simulink model "motor_idle"  (R2025b)
settings: Solver=ode45  StartTime=0.0  StopTime=10  MaxStep=0.02  RelTol=1e-3  AbsTol=1e-3
values from neighbouring files (symbols this model uses):
  B = 0.072    [parametros.m]
  Cd = 0.7    [parametros.m]
  emax = 1.8    [parametros.m]
  Hl = 44e6    (= 44000000)    [parametros.m]
  J = 0.25    [parametros.m]
  k1 = 1.44e5    (= 144000)    [parametros.m]
  k2 = 0.46    [parametros.m]
  k3 = 9.1e-4    (= 0.00091)    [parametros.m]
  k4 = 0.075    [parametros.m]
  kappa = 1.4    [parametros.m]
  kqueda = 0.001    [parametros.m]
  N0 = 800    [parametros.m]
  N_ciclo = 2    [parametros.m]
  nVol = 0.85    [parametros.m]
  omega0 = N0 * 2*pi/60    (= 83.7758040957)    [parametros.m]
  P_atm = 101325    [parametros.m]
  Pim0 = 40000    [parametros.m]
  R = 287    [parametros.m]
  S = 0.0814    [parametros.m]
  SA = 20    [parametros.m]
  SA_MBT = 25    [parametros.m]
  sigma0 = 14.7    [parametros.m]
  T_im = 300    [parametros.m]
  V = 0.0015    [parametros.m]
  V_d = 0.0013    [parametros.m]
settings Model: Creator=thiag  LastModifiedBy=thiag

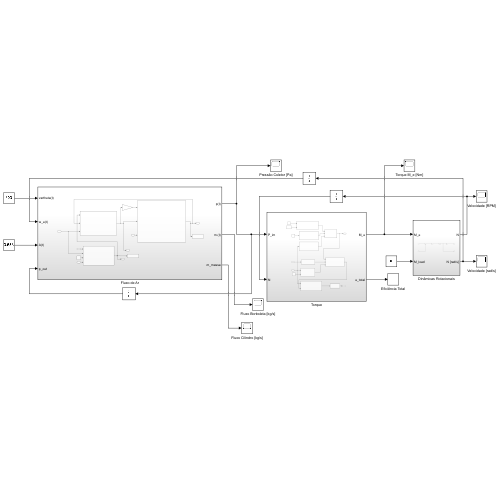
[thumbnail: Simulink's stored preview of the top-level diagram]
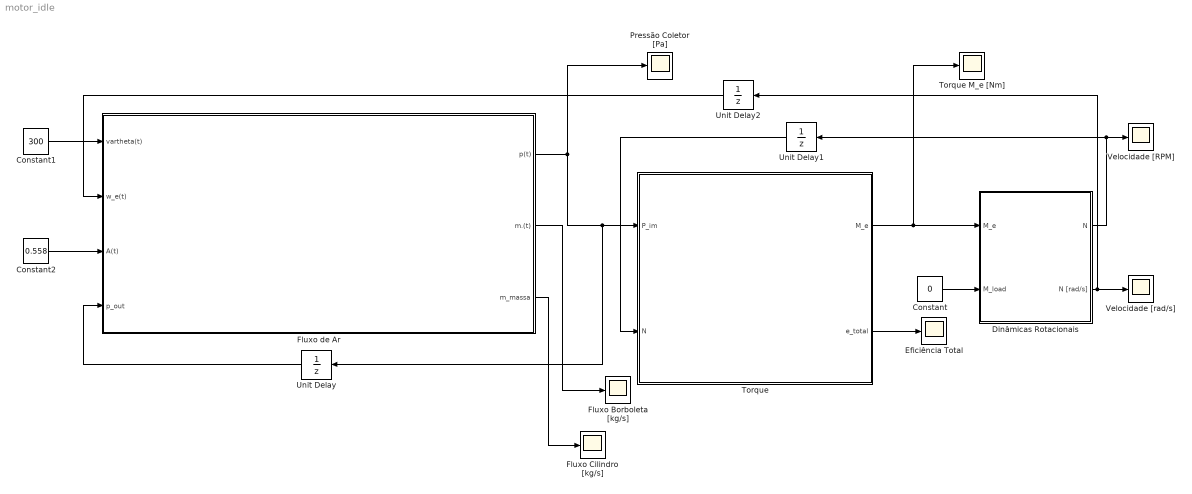
== system motor_idle ==
  Constant : Constant  Value=0
  Constant1 : Constant  Value=300
  Constant2 : Constant  Value=0.558
  Dinâmicas Rotacionais : Subsystem
  Eficiência Total : Scope
      settings: ActiveDisplayYMinimum=0.27237825090968576  ActiveDisplayYMaximum=0.32200698501713004  DataLoggingVariableName=ScopeData2
  Fluxo Borboleta [kg/s] : Scope
      settings: ActiveDisplayYMinimum=0.00082356518942528151  ActiveDisplayYMaximum=0.0010235651894252816  DataLoggingVariableName=ScopeData5
  Fluxo Cilindro [kg/s] : Scope
      settings: ActiveDisplayYMinimum=0.00036149983076327858  ActiveDisplayYMaximum=0.0037240393540282214  DataLoggingVariableName=ScopeData6
  Fluxo de Ar : Subsystem
  Pressão Coletor [Pa] : Scope
      settings: ActiveDisplayYMinimum=7090.5549569777586  ActiveDisplayYMaximum=43656.605004780249  DataLoggingVariableName=ScopeData3
  Torque : Subsystem
  Torque M_e [Nm] : Scope
      settings: ActiveDisplayYMinimum=-87.316847243549518  ActiveDisplayYMaximum=243.76291501335962  DataLoggingVariableName=ScopeData4
  Unit Delay : UnitDelay  InitialCondition=Pim0  SampleTime=0.02  HasFrameUpgradeWarning=on
  Unit Delay1 : UnitDelay  InitialCondition=N0  SampleTime=0.02  HasFrameUpgradeWarning=on
  Unit Delay2 : UnitDelay  InitialCondition=omega0  SampleTime=0.02  HasFrameUpgradeWarning=on
  Velocidade [RPM] : Scope
      settings: ActiveDisplayYMinimum=398.86041068334004  ActiveDisplayYMaximum=1697.6811601075797
  Velocidade [rad/s] : Scope
      settings: ActiveDisplayYMinimum=55.585400826373068  ActiveDisplayYMaximum=178.72399012064108
  wires:
  Dinâmicas Rotacionais/2(N [rad/s]) -> Velocidade [rad/s]/1, Unit Delay2/1
  Dinâmicas Rotacionais/1(N) -> Unit Delay1/1, Velocidade [RPM]/1
  Torque/2(e_total) -> Eficiência Total/1
  Torque/1(M_e) -> Torque M_e [Nm]/1, Dinâmicas Rotacionais/1(M_e)
  Fluxo de Ar/1(p(t)) -> Unit Delay/1, Torque/1(P_im), Pressão Coletor [Pa]/1
  Constant/1 -> Dinâmicas Rotacionais/2(M_load)
  Constant1/1 -> Fluxo de Ar/1(vartheta(t))
  Constant2/1 -> Fluxo de Ar/3(A(t))
  Fluxo de Ar/2(m.(t)) -> Fluxo Borboleta [kg/s]/1
  Fluxo de Ar/3(m_massa) -> Fluxo Cilindro [kg/s]/1
  Unit Delay/1 -> Fluxo de Ar/4(p_out)
  Unit Delay2/1 -> Fluxo de Ar/2(w_e(t))
  Unit Delay1/1 -> Torque/2(N)

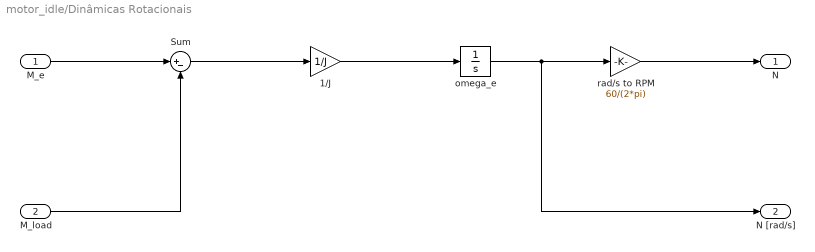
== system motor_idle/Dinâmicas Rotacionais ==
  M_e : Inport
  M_load : Inport  Port=2
  1/J : Gain  Gain=1/J
  Sum : Sum  Inputs=|+-
  omega_e : Integrator  InitialCondition=(N0*2*pi)/60
  rad/s to RPM : Gain  Gain=60/(2*pi)
  N : Outport
  N [rad/s] : Outport  Port=2
  wires:
  M_e/1 -> Sum/1
  M_load/1 -> Sum/2
  Sum/1 -> 1/J/1
  1/J/1 -> omega_e/1
  omega_e/1 -> N [rad/s]/1, rad/s to RPM/1
  rad/s to RPM/1 -> N/1

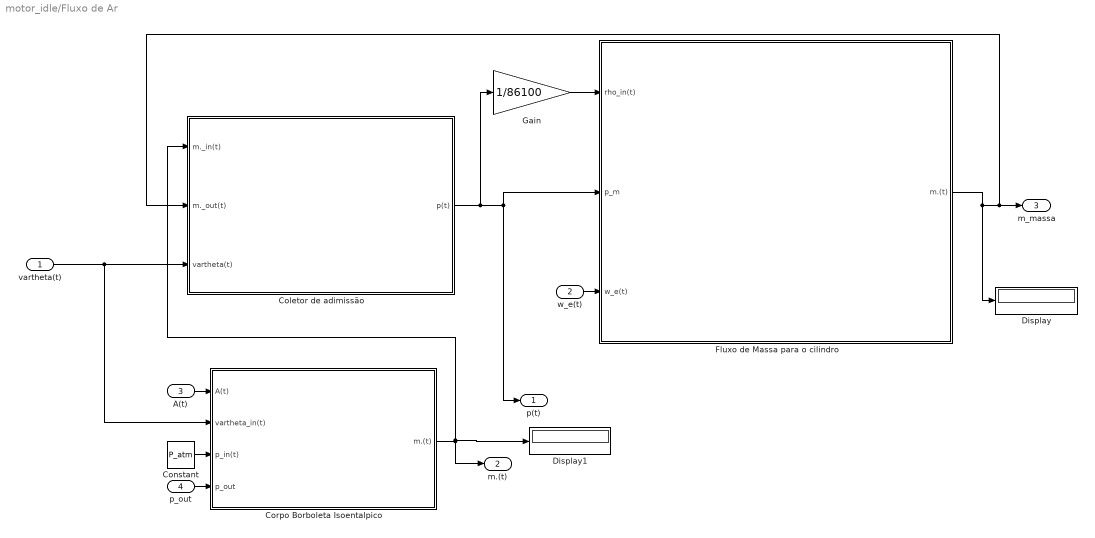
== system motor_idle/Fluxo de Ar ==
  vartheta(t) : Inport
  w_e(t) : Inport  Port=2
  A(t) : Inport  Port=3
  p_out : Inport  Port=4
  Coletor de adimissão : Subsystem
  Constant : Constant  Value=P_atm
  Corpo Borboleta Isoentalpico : Subsystem
  Display : Display
  Display1 : Display
  Fluxo de Massa para o cilindro : Subsystem
  Gain : Gain  Gain=1/86100
  p(t) : Outport
  m.(t) : Outport  Port=2
  m_massa : Outport  Port=3
  wires:
  Coletor de adimissão/1(p(t)) -> p(t)/1, Fluxo de Massa para o cilindro/2(p_m), Gain/1
  Constant/1 -> Corpo Borboleta Isoentalpico/3(p_in(t))
  Corpo Borboleta Isoentalpico/1(m.(t)) -> m.(t)/1, Display1/1, Coletor de adimissão/1(m._in(t))
  p_out/1 -> Corpo Borboleta Isoentalpico/4(p_out)
  w_e(t)/1 -> Fluxo de Massa para o cilindro/3(w_e(t))
  Fluxo de Massa para o cilindro/1(m.(t)) -> Display/1, m_massa/1, Coletor de adimissão/2(m._out(t))
  A(t)/1 -> Corpo Borboleta Isoentalpico/1(A(t))
  vartheta(t)/1 -> Corpo Borboleta Isoentalpico/2(vartheta_in(t)), Coletor de adimissão/3(vartheta(t))
  Gain/1 -> Fluxo de Massa para o cilindro/1(rho_in(t))

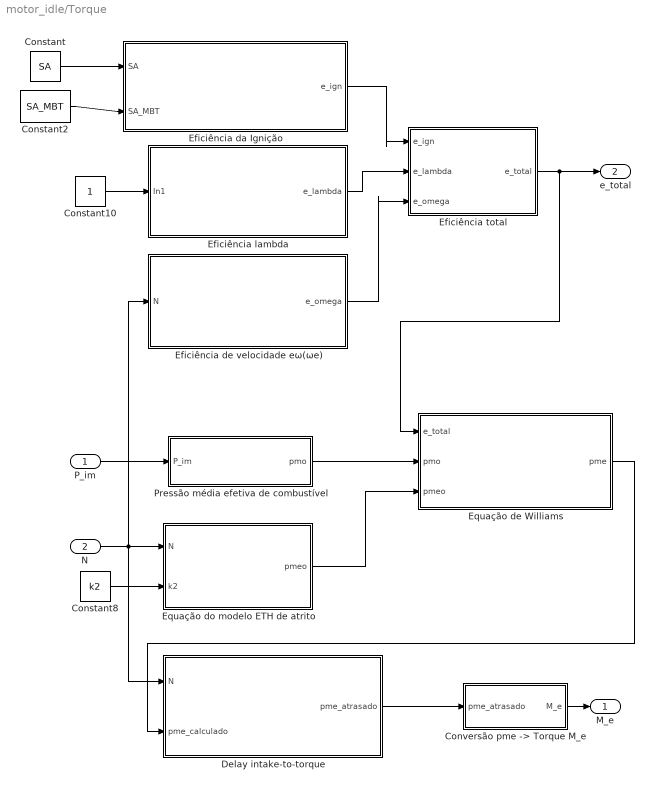
== system motor_idle/Torque ==
  P_im : Inport
  N : Inport  Port=2
  Constant : Constant  Value=SA
  Constant10 : Constant
  Constant2 : Constant  Value=SA_MBT
  Constant8 : Constant  Value=k2
  "Conversão pme -> Torque M_e" : Subsystem
  Delay intake-to-torque : Subsystem
  Eficiência da Ignição : Subsystem
  Eficiência de velocidade eω(ωe) : Subsystem
  Eficiência lambda : Subsystem
  Eficiência total : Subsystem
  Equação de Williams : Subsystem
  Equação do modelo ETH de atrito : Subsystem
  Pressão média efetiva de combustível : Subsystem
  M_e : Outport
  e_total : Outport  Port=2
  wires:
  N/1 -> Delay intake-to-torque/1(N), Eficiência de velocidade eω(ωe)/1(N), Equação do modelo ETH de atrito/1(N)
  Eficiência de velocidade eω(ωe)/1(e_omega) -> Eficiência total/3(e_omega)
  Constant/1 -> Eficiência da Ignição/1(SA)
  Equação do modelo ETH de atrito/1(pmeo) -> Equação de Williams/3(pmeo)
  Constant2/1 -> Eficiência da Ignição/2(SA_MBT)
  P_im/1 -> Pressão média efetiva de combustível/1(P_im)
  Equação de Williams/1(pme) -> Delay intake-to-torque/2(pme_calculado)
  Eficiência lambda/1(e_lambda) -> Eficiência total/2(e_lambda)
  Pressão média efetiva de combustível/1(pmo) -> Equação de Williams/2(pmo)
  Constant8/1 -> Equação do modelo ETH de atrito/2(k2)
  Constant10/1 -> Eficiência lambda/1(In1)
  Delay intake-to-torque/1(pme_atrasado) -> "Conversão pme -> Torque M_e"/1(pme_atrasado)
  Eficiência da Ignição/1(e_ign) -> Eficiência total/1(e_ign)
  Eficiência total/1(e_total) -> e_total/1, Equação de Williams/1(e_total)
  "Conversão pme -> Torque M_e"/1(M_e) -> M_e/1

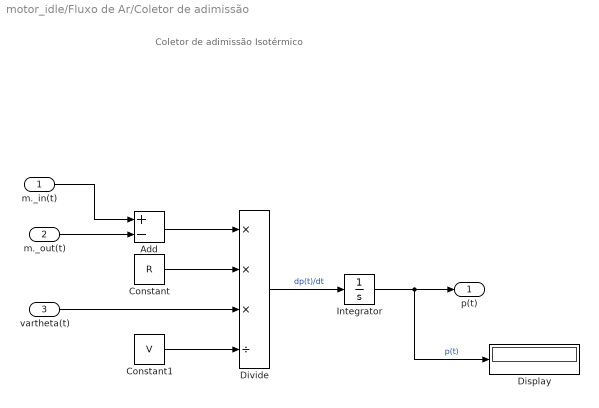
== system motor_idle/Fluxo de Ar/Coletor de adimissão ==
  note: Coletor de adimissão Isotérmico
  m._in(t) : Inport
  m._out(t) : Inport  Port=2
  vartheta(t) : Inport  Port=3
  Add : Sum  Inputs=+-
  Constant : Constant  Value=R
  Constant1 : Constant  Value=V
  Display : Display
  Divide : Product  Inputs=***/
  Integrator : Integrator  InitialCondition=Pim0
  p(t) : Outport
  wires:
  Add/1 -> Divide/1
  Constant/1 -> Divide/2
  m._in(t)/1 -> Add/1
  Divide/1 -> Integrator/1  "dp(t)/dt"
  Constant1/1 -> Divide/4
  m._out(t)/1 -> Add/2
  Integrator/1 -> Display/1, p(t)/1  "p(t)"
  vartheta(t)/1 -> Divide/3

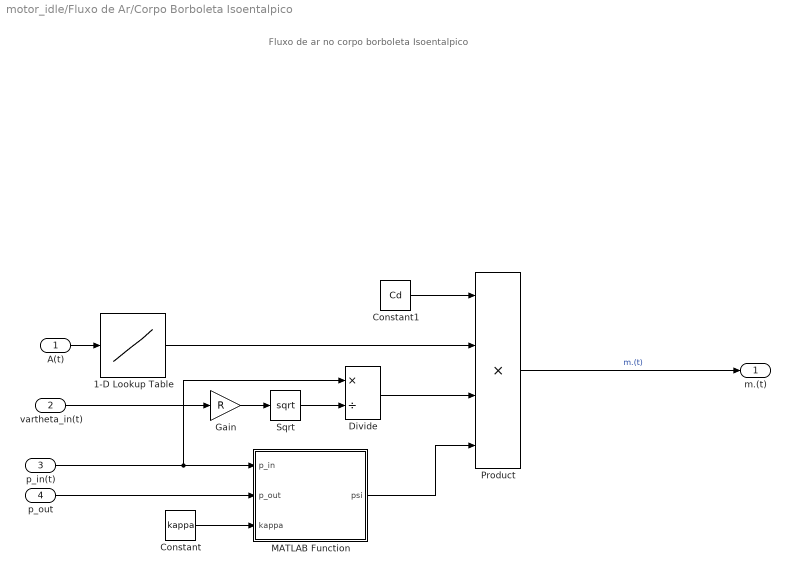
== system motor_idle/Fluxo de Ar/Corpo Borboleta Isoentalpico ==
  note: Fluxo de ar no corpo borboleta Isoentalpico
  A(t) : Inport
  vartheta_in(t) : Inport  Port=2
  p_in(t) : Inport  Port=3
  p_out : Inport  Port=4
  1-D Lookup Table : Lookup_n-D  NumberOfTableDimensions=1  BreakpointsForDimension1=[0, 5, 10, 20, 45, 90]  Table=[0, 5e-5, 1e-4, 2e-4, 3.5e-4, 5e-4]  InternalRulePriority=Speed  RndMeth=Simplest
  Constant : Constant  Value=kappa
  Constant1 : Constant  Value=Cd
  Divide : Product  Inputs=*/
  Gain : Gain  Gain=R
  MATLAB Function : MATLAB Function  TreatAsAtomicUnit=on
  Product : Product  Inputs=4
  Sqrt : Sqrt
  m.(t) : Outport
  wires:
  Constant/1 -> MATLAB Function/3(kappa)
  MATLAB Function/1(psi) -> Product/4
  p_in(t)/1 -> Divide/1, MATLAB Function/1(p_in)
  Sqrt/1 -> Divide/2
  Gain/1 -> Sqrt/1
  Divide/1 -> Product/3
  Constant1/1 -> Product/1
  Product/1 -> m.(t)/1  "m.(t)"
  vartheta_in(t)/1 -> Gain/1
  p_out/1 -> MATLAB Function/2(p_out)
  1-D Lookup Table/1 -> Product/2
  A(t)/1 -> 1-D Lookup Table/1

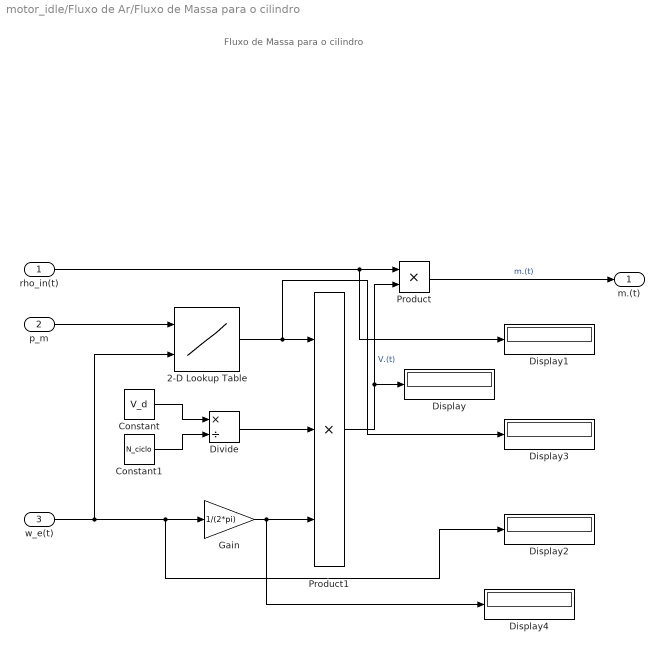
== system motor_idle/Fluxo de Ar/Fluxo de Massa para o cilindro ==
  note: Fluxo de Massa para o cilindro
  rho_in(t) : Inport
  p_m : Inport  Port=2
  w_e(t) : Inport  Port=3
  2-D Lookup Table : Lookup_n-D  BreakpointsForDimension1=[20000, 40000, 60000, 80000, 101325]  BreakpointsForDimension2=[52, 83, 105, 157, 209]  Table=[0.60 0.62 0.63 0.65 0.66; 0.75 0.78 0.80 0.82 0.83; 0.82 0.84 0.85 0.86 0.87; 0.85 0.86 0.87 0.88 0.89; 0.87 0.88 0.89 0.90 0.91]  InternalRulePriority=Speed  RndMeth=Simplest
      settings: InputPortMap=u0,u1
  Constant : Constant  Value=V_d
  Constant1 : Constant  Value=N_ciclo
  Display{,1..4} (5 alike) : Display
  Divide : Product  Inputs=*/
  Gain : Gain  Gain=1/(2*pi)
  Product : Product
  Product1 : Product  Inputs=3
  m.(t) : Outport
  wires:
  rho_in(t)/1 -> Display1/1, Product/1
  Product1/1 -> Display/1, Product/2  "V.(t)"
  p_m/1 -> 2-D Lookup Table/1
  Constant1/1 -> Divide/2
  Constant/1 -> Divide/1
  Gain/1 -> Display4/1, Product1/3
  Divide/1 -> Product1/2
  2-D Lookup Table/1 -> Display3/1, Product1/1
  Product/1 -> m.(t)/1  "m.(t)"
  w_e(t)/1 -> 2-D Lookup Table/2, Display2/1, Gain/1

== system motor_idle/Torque/Conversão pme -> Torque M_e ==
  pme_atrasado : Inport
  Gain7 : Gain  Gain=V_d/4*pi
  M_e : Outport
  wires:
  Gain7/1 -> M_e/1
  pme_atrasado/1 -> Gain7/1

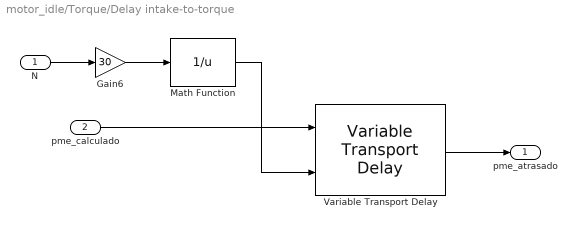
== system motor_idle/Torque/Delay intake-to-torque ==
  N : Inport
  pme_calculado : Inport  Port=2
  Gain6 : Gain  Gain=30
  Math Function : Math  Operator=reciprocal
  Variable Transport Delay : VariableTransportDelay  VariableDelayType=Variable transport delay  MaximumDelay=0.1  MaximumPoints=8192
  pme_atrasado : Outport
  wires:
  pme_calculado/1 -> Variable Transport Delay/1
  N/1 -> Gain6/1
  Gain6/1 -> Math Function/1
  Math Function/1 -> Variable Transport Delay/2
  Variable Transport Delay/1 -> pme_atrasado/1

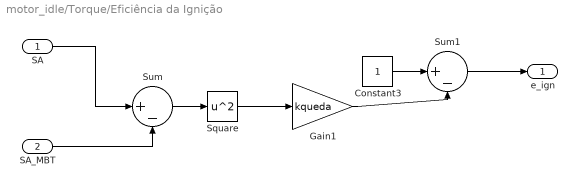
== system motor_idle/Torque/Eficiência da Ignição ==
  SA : Inport
  SA_MBT : Inport  Port=2
  Constant3 : Constant
  Gain1 : Gain  Gain=kqueda
  Square : Math  Operator=square
  Sum : Sum  Inputs=|+-
  Sum1 : Sum  Inputs=|+-
  e_ign : Outport
  wires:
  Gain1/1 -> Sum1/2
  Sum1/1 -> e_ign/1
  Constant3/1 -> Sum1/1
  SA/1 -> Sum/1
  SA_MBT/1 -> Sum/2
  Square/1 -> Gain1/1
  Sum/1 -> Square/1

== system motor_idle/Torque/Eficiência de velocidade eω(ωe) ==
  N : Inport
  1-D Lookup Table1 : Lookup_n-D  NumberOfTableDimensions=1  BreakpointsForDimension1="[52,  83,  105, 157, 209, 262, 314, 419, 524, 628]"  Table=[0.28, 0.30, 0.31, 0.33, 0.34, 0.35, 0.35, 0.34, 0.32, 0.29]  InternalRulePriority=Speed  RndMeth=Simplest
  Gain2 : Gain  Gain=(2*pi)/60
  e_omega : Outport
  wires:
  N/1 -> Gain2/1
  1-D Lookup Table1/1 -> e_omega/1
  Gain2/1 -> 1-D Lookup Table1/1

== system motor_idle/Torque/Eficiência lambda ==
  In1 : Inport
  1-D Lookup Table : Lookup_n-D  NumberOfTableDimensions=1  BreakpointsForDimension1=[0.70, 0.80, 0.90, 0.95, 1.00, 1.03, 1.10, 1.30]  Table=[0.59, 0.72, 0.86, 0.93, 0.98, 1.00, 1.00, 1.00]  InternalRulePriority=Speed  RndMeth=Simplest
  e_lambda : Outport
  wires:
  In1/1 -> 1-D Lookup Table/1
  1-D Lookup Table/1 -> e_lambda/1

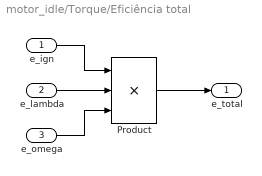
== system motor_idle/Torque/Eficiência total ==
  e_ign : Inport
  e_lambda : Inport  Port=2
  e_omega : Inport  Port=3
  Product : Product  Inputs=3
  e_total : Outport
  wires:
  Product/1 -> e_total/1
  e_omega/1 -> Product/3
  e_lambda/1 -> Product/2
  e_ign/1 -> Product/1

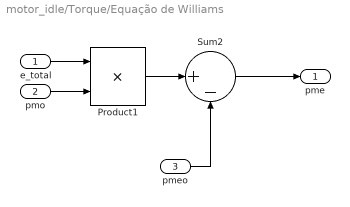
== system motor_idle/Torque/Equação de Williams ==
  e_total : Inport
  pmo : Inport  Port=2
  pmeo : Inport  Port=3
  Product1 : Product
  Sum2 : Sum  Inputs=|+-
  pme : Outport
  wires:
  Product1/1 -> Sum2/1
  Sum2/1 -> pme/1
  pmeo/1 -> Sum2/2
  e_total/1 -> Product1/1
  pmo/1 -> Product1/2

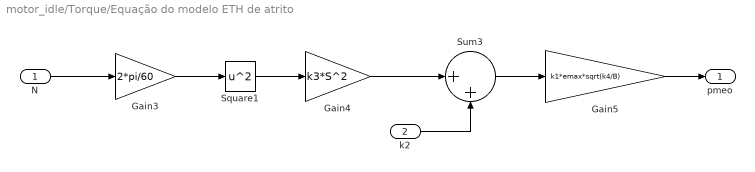
== system motor_idle/Torque/Equação do modelo ETH de atrito ==
  N : Inport
  k2 : Inport  Port=2
  Gain3 : Gain  Gain=2*pi/60
  Gain4 : Gain  Gain=k3*S^2
  Gain5 : Gain  Gain=k1*emax*sqrt(k4/B)
  Square1 : Math  Operator=square
  Sum3 : Sum  Inputs=|++
  pmeo : Outport
  wires:
  Gain4/1 -> Sum3/1
  Gain5/1 -> pmeo/1
  Gain3/1 -> Square1/1
  k2/1 -> Sum3/2
  N/1 -> Gain3/1
  Sum3/1 -> Gain5/1
  Square1/1 -> Gain4/1

== system motor_idle/Torque/Pressão média efetiva de combustível ==
  P_im : Inport
  Gain : Gain  Gain=nVol*Hl/(sigma0*R*T_im)
  pmo : Outport
  wires:
  P_im/1 -> Gain/1
  Gain/1 -> pmo/1

== matlab function motor_idle/Fluxo de Ar/Corpo Borboleta Isoentalpico/MATLAB Function ==
  data: p_in input; psi output; p_out input; kappa input
function psi = psiFcn(p_in, p_out, kappa)
%psiFcn Função de fluxo Ψ
%   Detailed explanation goes here
arguments (Input)
    p_in;       %pressão de entrada
    p_out;      %pressão de saida;
    kappa;
end

arguments (Output)
    psi
end
    p_cr = p_in * (2/(kappa+1))^(kappa/(kappa-1));
    if p_out < p_cr
        % Fluxo Sônico (Choked)
        psi = sqrt(kappa * (2/(kappa+1))^((kappa+1)/(kappa-1)));
    else
        % Fluxo Subsônico
        term1 = (p_out/p_in)^(1/kappa);
        term2 = sqrt((2*kappa)/(kappa-1) * (1 - (p_out/p_in)^((kappa-1)/kappa)));
        psi = term1 * term2;
    end
end
